simulink model "ROPOD_4Wheel_TdistZMPC_cntr_EC"  (R2017b)
settings: Solver=ode1  StartTime=0.0  StopTime=Tfinal  FixedStep=Ts  RelTol=1e-3  EnableMultiTasking=on
PreLoadFcn:
  | init_model
InitFcn:
  | init_model
values from neighbouring files (symbols this model uses):
  b_cx = 70.26    [RoPod_parameters.mat]
  b_cy = 36.5    [RoPod_parameters.mat]
  FFtheta_intia = 0    [init_model.m]
  FFxy_mass = 80    [init_model.m]
  I_fhz_dtheta_cntr = 0.5    [init_model.m]
  I_fhz_dvarphi_cntr = 0    [init_model.m]
  I_fhz_dxdy_cntr = 0.25    [init_model.m]
  k_cx = 4300    [RoPod_parameters.mat]
  k_cy = 4489    [RoPod_parameters.mat]
  K_gain_dtheta_cntr = 150    [init_model.m]
  K_gain_dvarphi_cntr = 0.05    [init_model.m]
  K_gain_dxdy_cntr = 200    [init_model.m]
  LL_wp_fhz_dtheta_cntr = 20    [init_model.m]
  LL_wp_fhz_dvarphi_cntr = 20    [init_model.m]
  LL_wp_fhz_dxdy_cntr = 20    [init_model.m]
  LL_wz_fhz_dtheta_cntr = 20    [init_model.m]
  LL_wz_fhz_dvarphi_cntr = 2    [init_model.m]
  LL_wz_fhz_dxdy_cntr = 20    [init_model.m]
  LPF_fhz_dtheta_cntr = 100    [init_model.m]
  LPF_fhz_dvarphi_cntr = 100    [init_model.m]
  LPF_fhz_dxdy_cntr = 100    [init_model.m]
  max_hw_tau = 7.0    (= 7)    [init_model.m]
  max_ropod_acc_theta = 1.6    [init_model.m]
  max_ropod_acc_xy = 1.0    (= 1)    [init_model.m]
  max_ropod_vel_theta = 1.6    [init_model.m]
  max_ropod_vel_xy = 1.0    (= 1)    [init_model.m]
  max_sw_current = 10    [init_model.m]
  Nwheels = 4    [init_model.m]
  pivot_offs_sws = [2.21 1.873 2.001 3.508]    [init_model.m]
  SW_COM1_ENABLE1 = hex2dec('0001')    [init_model.m]
  SW_COM1_ENABLE2 = hex2dec('0002')    [init_model.m]
  SW_COM1_MODE_TORQUE = bitshift(hex2dec('0000'),2)    [init_model.m]
  SW_COM1_MODE_VELOCITY = bitshift(hex2dec('0002'),2)    [init_model.m]
  SW_COM1_USE_TS = hex2dec('8000')    [init_model.m]
  sw_tau_2_curr = 1/motor_physical_parameters.torqueconstant.value    [init_model.m]
  Taucompfactor = 2.0    (= 2)    [init_model.m]
  Tinit = 1*Tslot    [init_model.m]
  Ts = 0.001    [init_model.m]
  Ts_MPC = 0.001    [init_model.m]
  xA = [1 -1 0 0 0 0 0.0206696424966 -0.0206696424966 0 0 0.0298227588181 -0.0298227588181 ... (4080 elements, 102x40)]    [ZMPCx_parameters.mat]
  xBd_dis = [1.12932348493e-06 0.000225071897401 0 0]    [ZMPCx_parameters.mat]
  xF = [0 0 0 0 0 0 0 0 0 0 0 0 ... (80 elements, 20x4)]    [ZMPCx_parameters.mat]
  xH = [20 0 0 0 0 0 0 0 0 0 0 0 ... (1600 elements, 40x40)]    [ZMPCx_parameters.mat]
  xPhi = [0.995143909015 -0.967809158823 0 0 0.980727027327 -1.91066813489 0 0 0.957042868744 -2.81984596436 0 0 ... (320 elements, 80x4)]    [ZMPCx_parameters.mat]
  xrho = 144000    [ZMPCx_parameters.mat]
  xW = [0 0 -4300 4300 0 0 -4211.12053726 4211.12053726 0 0 -4082.88267435 4082.88267435 ... (328 elements, 82x4)]    [ZMPCx_parameters.mat]
  yA = [1 -1 0 0 0 0 0.0146537039222 -0.0146537039222 0 0 0.0255124036215 -0.0255124036215 ... (4080 elements, 102x40)]    [ZMPCy_parameters.mat]
  yBd_dis = [1.24492522358e-06 0.000248362591603 0 0]    [ZMPCy_parameters.mat]
  yF = [0.00191047141222 0.00156448969707 0.00119761396088 0.000813779538874 0.00041715000072 1.20724055612e-05 -0.00039696993291 -0.000805406662726 -0.00120863105559 -0.00160205155743 -0.00198114365531 -0.00234150147928 ... (80 elements, 20x4)]    [ZMPCy_parameters.mat]
  yH = [2.00000002801 0 2.31602594113e-08 0 1.80085634996e-08 0 1.26053094289e-08 0 7.00898668547e-09 0 1.2808124932e-09 0 ... (1600 elements, 40x40)]    [ZMPCy_parameters.mat]
  yPhi = [0.994411530671 -1.11489967371 0 0 0.977778317439 -2.20691845877 0 0 0.950389393786 -3.2640842851 0 0 ... (320 elements, 80x4)]    [ZMPCy_parameters.mat]
  yrho = 10000    [ZMPCy_parameters.mat]
  yW = [0 0 -4489 4489 0 0 -4423.21952309 4423.21952309 0 0 -4308.69434324 4308.69434324 ... (328 elements, 82x4)]    [ZMPCy_parameters.mat]
undefined symbols (not defined in the file or in its folder): DiscIntNeverNeededParam, Fd_max, Fd_min, Fr_max, Fr_min, ropod_kinmodel_param
libraries: cstblocks x85, simulink x41, SOEM_EtherCAT_Lib x5
(part 5 of 5)

== stateflow chart ROPOD_4Wheel_TdistZMPC_cntr_EC/Non-ROS Ropod Controller/State machine1/Chart ==
  state Mode1_Operation_mode
    state Collision_with_object
      entry: state = 2
      state Interaction_front
        entry: ZMPC_x = 1
        entry: ZMPCx_Fd_min = 0
        entry: ZMPCx_Fd_max = Fd_max
      state Interaction_left_side
        entry: ZMPC_y = 1
        entry: ZMPCy_Fd_min = 0
        entry: ZMPCy_Fd_max = Fd_max
      state Interaction_right_side
        entry: ZMPC_y = 1
        entry: ZMPCy_Fd_min = -Fd_max
        entry: ZMPCy_Fd_max = 0
      state No_interaction
        entry: ZMPC_x = 0
        entry: ZMPC_y = 0
        entry: ZMPC_o = 0
      state Interaction_back
        entry: ZMPC_x = 1
        entry: ZMPCx_Fd_min = -Fd_max
        entry: ZMPCx_Fd_max = 0
      (default) -> Interaction_front
      Interaction_front -> Mode1_Operation_mode.Collision_with_object.No_interaction : [interaction_force_x < (Fd_min-2) ]
      Mode1_Operation_mode.Collision_with_object.No_interaction -> Interaction_front [order 3] : [interaction_force_x > (Fd_min+2)]
      Mode1_Operation_mode.Collision_with_object.No_interaction -> Mode1_Operation_mode.Collision_with_object.Interaction_left_side [order 1] : [interaction_force_y > (Fd_min+2)]
      Mode1_Operation_mode.Collision_with_object.No_interaction -> Mode1_Operation_mode.Collision_with_object.Interaction_right_side [order 2] : [interaction_force_y < -(Fd_min+2)]
      Mode1_Operation_mode.Collision_with_object.Interaction_right_side -> Mode1_Operation_mode.Collision_with_object.No_interaction : [interaction_force_y > -(Fd_min-2)]
      Mode1_Operation_mode.Collision_with_object.Interaction_left_side -> Mode1_Operation_mode.Collision_with_object.No_interaction : [interaction_force_y < (Fd_min-2) ]
      Mode1_Operation_mode.Collision_with_object.No_interaction -> Interaction_back [order 4] : [interaction_force_x < -(Fd_min+2)]
      Interaction_back -> Mode1_Operation_mode.Collision_with_object.No_interaction : [interaction_force_x > -(Fd_min-2)]
    state Interaction_left_side
      entry: state = 3
      entry: ZMPC_y = 1
      entry: ZMPCy_Fd_min = 0
      entry: ZMPCy_Fd_max = Fd_max
    state Interaction_right_side
      entry: state = 3
      entry: ZMPC_y = 1
      entry: ZMPCy_Fd_min = -Fd_max
      entry: ZMPCy_Fd_max = 0
    state No_interaction
      entry: state = 1
      entry: ZMPC_x = 0
      entry: ZMPC_y = 0
      entry: ZMPC_o = 0
    Mode1_Operation_mode.Interaction_left_side -> Collision_with_object [order 2] : [interaction_force_x > Fd_min]
    Mode1_Operation_mode.No_interaction -> Collision_with_object [order 1] : [interaction_force_x > Fd_min]
    Mode1_Operation_mode.Interaction_right_side -> Collision_with_object [order 2] : [interaction_force_x > Fd_min]
    Mode1_Operation_mode.No_interaction -> Mode1_Operation_mode.Interaction_left_side [order 2] : [interaction_force_y > (Fd_min+2)]
    Mode1_Operation_mode.No_interaction -> Mode1_Operation_mode.Interaction_right_side [order 3] : [interaction_force_y < -(Fd_min+2)]
    Mode1_Operation_mode.Interaction_right_side -> Mode1_Operation_mode.No_interaction [order 1] : [interaction_force_y > -(Fd_min-2)]
    Mode1_Operation_mode.Interaction_left_side -> Mode1_Operation_mode.No_interaction [order 1] : [interaction_force_y < (Fd_min-2) ]
    (default) -> Mode1_Operation_mode.No_interaction
  state Mode4_Connect_to_cart
    state Connect_to_cart
      entry: ZMPC_x = 0
      entry: ZMPC_y = 0
      entry: ZMPC_o = 0
    state Hold_contact_with_cart
      entry: state = 4
      entry: ZMPC_x = 1
      entry: ZMPC_o = 1
      entry: ZMPCx_Fd_min = -Fd_max
      entry: ZMPCx_Fd_max = -Fd_min
    (default) -> Connect_to_cart
    Hold_contact_with_cart -> Connect_to_cart : [interaction_force_x > -(Fd_min-7)]
    Connect_to_cart -> Hold_contact_with_cart : [interaction_force_x < -(Fd_min+2)]
  state Velocity_control
    entry: state = 0
    entry: ZMPC_x = 0
    entry: ZMPC_y = 0
    entry: ZMPC_o = 0
    entry: ZMPCx_Fd_min = 0
    entry: ZMPCx_Fd_max = Fd_max
    entry: ZMPCy_Fd_min = 0
    entry: ZMPCy_Fd_max = Fd_max
  (default) -> Velocity_control
  Velocity_control -> Mode1_Operation_mode : [mode == 1]
  Mode1_Operation_mode -> Mode4_Connect_to_cart : [mode == 4]
  Collision_with_object -> Velocity_control : [mode == 0]
  Mode4_Connect_to_cart -> Mode1_Operation_mode : [mode == 1]
  data: interaction_force_x input; ZMPC_x output; ZMPC_y output; ZMPC_o output; interaction_force_y input; Fd_min input; ZMPCx_Fd_min output; ZMPCy_Fd_min output; Fd_max input; ZMPCx_Fd_max output; ZMPCy_Fd_max output; state output; mode input

== matlab function ROPOD_4Wheel_TdistZMPC_cntr_EC/Non-ROS Ropod Controller/platform vel cntr/Bumper Interaction Controller/Bumper_system/cal1/Calibration1 ==
  data: angle input; cal_angle output; sample input; i output; data input; data_out output
function [cal_angle, i, data_out]= fcn(angle,sample,data)
cal_start_sample = 1000;
cal_end_sample = 2000;

if sample > cal_start_sample && sample <= cal_end_sample
    data_out = data+angle; 
    cal_angle = angle;
else
    correction = data/(cal_end_sample - cal_start_sample);
    cal_angle = angle-correction;
    data_out = data;
end

i = sample+1;

== matlab function ROPOD_4Wheel_TdistZMPC_cntr_EC/Non-ROS Ropod Controller/platform vel cntr/Bumper Interaction Controller/Bumper_system/cal2/Calibration1 ==
  data: angle input; cal_angle output; sample input; i output; data input; data_out output
function [cal_angle, i, data_out]= fcn(angle,sample,data)
cal_start_sample = 1000;
cal_end_sample = 2000;

if sample > cal_start_sample && sample <= cal_end_sample
    data_out = data+angle; 
    cal_angle = angle;
else
    correction = data/(cal_end_sample - cal_start_sample);
    cal_angle = angle-correction;
    data_out = data;
end

i = sample+1;

== matlab function ROPOD_4Wheel_TdistZMPC_cntr_EC/Non-ROS Ropod Controller/platform vel cntr/Bumper Interaction Controller/Bumper_system/cal3/Calibration1 ==
  data: angle input; cal_angle output; sample input; i output; data input; data_out output
function [cal_angle, i, data_out]= fcn(angle,sample,data)
cal_start_sample = 1000;
cal_end_sample = 2000;

if sample > cal_start_sample && sample <= cal_end_sample
    data_out = data+angle; 
    cal_angle = angle;
else
    correction = data/(cal_end_sample - cal_start_sample);
    cal_angle = angle-correction;
    data_out = data;
end

i = sample+1;

== matlab function ROPOD_4Wheel_TdistZMPC_cntr_EC/Non-ROS Ropod Controller/platform vel cntr/Bumper Interaction Controller/Bumper_system/cal4/Calibration1 ==
  data: angle input; cal_angle output; sample input; i output; data input; data_out output
function [cal_angle, i, data_out]= fcn(angle,sample,data)
cal_start_sample = 1000;
cal_end_sample = 2000;

if sample > cal_start_sample && sample <= cal_end_sample
    data_out = data+angle; 
    cal_angle = angle;
else
    correction = data/(cal_end_sample - cal_start_sample);
    cal_angle = angle-correction;
    data_out = data;
end

i = sample+1;

== matlab function ROPOD_4Wheel_TdistZMPC_cntr_EC/Non-ROS Ropod Controller/platform vel cntr/Bumper Interaction Controller/Bumper_system/cal5/Calibration1 ==
  data: angle input; cal_angle output; sample input; i output; data input; data_out output
function [cal_angle, i, data_out]= fcn(angle,sample,data)
cal_start_sample = 1000;
cal_end_sample = 2000;

if sample > cal_start_sample && sample <= cal_end_sample
    data_out = data+angle; 
    cal_angle = angle;
else
    correction = data/(cal_end_sample - cal_start_sample);
    cal_angle = angle-correction;
    data_out = data;
end

i = sample+1;

== matlab function ROPOD_4Wheel_TdistZMPC_cntr_EC/Non-ROS Ropod Controller/platform vel cntr/Bumper Interaction Controller/Bumper_system/cal6/Calibration1 ==
  data: angle input; cal_angle output; sample input; i output; data input; data_out output
function [cal_angle, i, data_out]= fcn(angle,sample,data)
cal_start_sample = 1000;
cal_end_sample = 2000;

if sample > cal_start_sample && sample <= cal_end_sample
    data_out = data+angle; 
    cal_angle = angle;
else
    correction = data/(cal_end_sample - cal_start_sample);
    cal_angle = angle-correction;
    data_out = data;
end

i = sample+1;

== matlab function ROPOD_4Wheel_TdistZMPC_cntr_EC/Non-ROS Ropod Controller/platform vel cntr/Bumper Interaction Controller/Bumper_system/cal7/Calibration1 ==
  data: angle input; cal_angle output; sample input; i output; data input; data_out output
function [cal_angle, i, data_out]= fcn(angle,sample,data)
cal_start_sample = 1000;
cal_end_sample = 2000;

if sample > cal_start_sample && sample <= cal_end_sample
    data_out = data+angle; 
    cal_angle = angle;
else
    correction = data/(cal_end_sample - cal_start_sample);
    cal_angle = angle-correction;
    data_out = data;
end

i = sample+1;

== stateflow chart ROPOD_4Wheel_TdistZMPC_cntr_EC/joystick_velocitie_sp/Chart ==
  state init
    entry: velocity_sp = [0; 0; 0]
  state Wait_for_joystick_command
    entry: mode = 0
    entry: velocity_sp = [0; 0; 0]
  state idle [commented out]
    entry: mode = 0
  state Move_right
    entry: velocity_sp = [0; -0.4; 0]
  state Rotate_left
    entry: velocity_sp = [0; 0; 0.4]
  state Rotate_right
    entry: velocity_sp = [0; 0; -0.4]
  state Move_back
    entry: mode = 1
  state Move_backward
    entry: velocity_sp = [-0.4; 0; 0]
  state Move_left
    entry: velocity_sp = [0; 0.4; 0]
  state Move_forward
    entry: mode = 1
    entry: velocity_sp = [0.4; 0; 0]
  state Connect_to_cart
    entry: connected_to_cart = 0
    entry: mode = 4
    entry: velocity_sp = [-0.3; 0; 0]
  state Connected_to_cart
    entry: velocity_sp = [0; 0; 0]
    entry: connected_to_cart = 1
  (default) -> init
  init -> Wait_for_joystick_command : after(3,sec)
  Wait_for_joystick_command -> idle [commented out] : [robot_speed(1) < 0.02 && robot_speed(1) > -0.02 && robot_speed(2) < 0.02 && robot_speed(2) > -0.02 && robot_speed(3) < 0.02 && robot_speed(3) > -0.02]
  idle -> Wait_for_joystick_command [commented out] : [joystick ~= 0]
  Wait_for_joystick_command -> Move_forward [order 3] : [joystick == 1]
  Move_forward -> Wait_for_joystick_command : [joystick ~= 1]
  Wait_for_joystick_command -> Move_backward [order 2] : [joystick == 2]
  Move_backward -> Wait_for_joystick_command : [joystick ~= 2]
  Wait_for_joystick_command -> Move_left [order 6] : [joystick == 3]
  Move_left -> Wait_for_joystick_command : [joystick ~= 3]
  Wait_for_joystick_command -> Move_right [order 5] : [joystick == 4]
  Move_right -> Wait_for_joystick_command : [joystick ~= 4]
  Rotate_left -> Wait_for_joystick_command : [joystick ~= 8]
  Wait_for_joystick_command -> Rotate_left [order 7] : [joystick == 8]
  Rotate_right -> Wait_for_joystick_command : [joystick ~= 9]
  Wait_for_joystick_command -> Rotate_right [order 4] : [joystick == 9]
  Connected_to_cart -> Wait_for_joystick_command
  Move_back -> Wait_for_joystick_command [order 1] : [joystick ~= 12]
  Wait_for_joystick_command -> Move_back [order 1] : [joystick == 12]
  Move_back -> Connect_to_cart [order 2] : [after(0.1,sec)]
  Connect_to_cart -> Connected_to_cart : [Fx_Fy_Tx_Ty(1) > 30 && joystick ~= 12]
  data: joystick input; velocity_sp output; robot_speed input; mode output; Fx_Fy_Tx_Ty input; connected_to_cart output

== matlab function ROPOD_4Wheel_TdistZMPC_cntr_EC/Non-ROS Ropod Controller/platform vel cntr/Bumper Interaction Controller/Bumper_system/cal8/Calibration1 ==
  data: angle input; cal_angle output; sample input; i output; data input; data_out output
function [cal_angle, i, data_out]= fcn(angle,sample,data)
cal_start_sample = 1000;
cal_end_sample = 2000;

if sample > cal_start_sample && sample <= cal_end_sample
    data_out = data+angle; 
    cal_angle = angle;
else
    correction = data/(cal_end_sample - cal_start_sample);
    cal_angle = angle-correction;
    data_out = data;
end

i = sample+1;

== matlab function ROPOD_4Wheel_TdistZMPC_cntr_EC/Non-ROS Ropod Controller/platform vel cntr/Bumper Interaction Controller/Bumper_system/speed deflection angle calculation X+ ==
  data: s_data input; Total_deflection output; Total_speed output; max_angle output
function [Total_deflection, Total_speed, max_angle] = Sensor_data(s_data)
% s_data is the sensor data
% s_data(1:4) = deflection in m
% s_data(5:8) = speed in m/s

% Parameters

%               V end-effector V            %
%-------------------------------------------%
% .            .             .            . %
% .            .             .            . %
%_I_          _I_           _I_          _I_%
% <     d1    ><     d2     ><      d3    > %
% x1          x2            x3           x4 %

d1 = 164; %mm
d2 = 164; %mm 
d3 = 164; %mm
dx = s_data(1:4); %deflection in m
dx_dot = s_data(5:8); %speed in m/s


% Deflection and speed in x direction
Total_deflection = sum(dx);
Total_speed = sum(dx_dot);


% Angle of the end-effector
angle_12 = atan((dx(1)-dx(2))/(d1));
angle_23 = atan((dx(2)-dx(3))/(d2));
angle_34 = atan((dx(3)-dx(4))/(d3));
angle_14 = atan((dx(1)-dx(4))/(d1+d2+d3));
angle = max([angle_12, angle_23, angle_34, angle_14]);
max_angle = rad2deg(angle);

end

== matlab function ROPOD_4Wheel_TdistZMPC_cntr_EC/Non-ROS Ropod Controller/platform vel cntr/Bumper Interaction Controller/Bumper_system/speed deflection angle calculation X- ==
  data: s_data input; Total_deflection output; Total_speed output; max_angle output
function [Total_deflection, Total_speed, max_angle] = Sensor_data(s_data)
% s_data is the sensor data
% s_data(1:4) = deflection in m
% s_data(5:8) = speed in m/s

% Parameters

%               V end-effector V            %
%-------------------------------------------%
% .            .             .            . %
% .            .             .            . %
%_I_          _I_           _I_          _I_%
% <     d1    ><     d2     ><      d3    > %
% x1          x2            x3           x4 %

d1 = 164; %mm
d2 = 164; %mm 
d3 = 164; %mm
dx = s_data(1:4); %deflection in m
dx_dot = s_data(5:8); %speed in m/s


% Deflection and speed in x direction
Total_deflection = sum(dx);
Total_speed = sum(dx_dot);


% Angle of the end-effector
angle_12 = atan((dx(1)-dx(2))/(d1));
angle_23 = atan((dx(2)-dx(3))/(d2));
angle_34 = atan((dx(3)-dx(4))/(d3));
angle_14 = atan((dx(1)-dx(4))/(d1+d2+d3));
angle = max([angle_12, angle_23, angle_34, angle_14]);
max_angle = rad2deg(angle);

end

== matlab function ROPOD_4Wheel_TdistZMPC_cntr_EC/Non-ROS Ropod Controller/platform vel cntr/Bumper Interaction Controller/Bumper_system/speed deflection angle calculation Y+ ==
  data: s_data input; Total_deflection output; Total_speed output; max_angle output
function [Total_deflection, Total_speed, max_angle] = Sensor_data(s_data)
% s_data is the sensor data
% s_data(1:4) = deflection in m
% s_data(5:8) = speed in m/s

% Parameters

%               V end-effector V            %
%-------------------------------------------%
% .            .             .            . %
% .            .             .            . %
%_I_          _I_           _I_          _I_%
% <     d1    ><     d2     ><      d3    > %
% x1          x2            x3           x4 %

d1 = 164; %mm
d2 = 164; %mm 
d3 = 164; %mm
dx = s_data(1:4); %deflection in m
dx_dot = s_data(5:8); %speed in m/s


% Deflection and speed in x direction
Total_deflection = sum(dx);
Total_speed = sum(dx_dot);


% Angle of the end-effector
angle_12 = atan((dx(1)-dx(2))/(d1));
angle_23 = atan((dx(2)-dx(3))/(d2));
angle_34 = atan((dx(3)-dx(4))/(d3));
angle_14 = atan((dx(1)-dx(4))/(d1+d2+d3));
angle = max([angle_12, angle_23, angle_34, angle_14]);
max_angle = rad2deg(angle);

end

== matlab function ROPOD_4Wheel_TdistZMPC_cntr_EC/Non-ROS Ropod Controller/platform vel cntr/Bumper Interaction Controller/Bumper_system/speed deflection angle calculation Y- ==
  data: s_data input; Total_deflection output; Total_speed output; max_angle output
function [Total_deflection, Total_speed, max_angle] = Sensor_data(s_data)
% s_data is the sensor data
% s_data(1:4) = deflection in m
% s_data(5:8) = speed in m/s

% Parameters

%               V end-effector V            %
%-------------------------------------------%
% .            .             .            . %
% .            .             .            . %
%_I_          _I_           _I_          _I_%
% <     d1    ><     d2     ><      d3    > %
% x1          x2            x3           x4 %

d1 = 164; %mm
d2 = 164; %mm 
d3 = 164; %mm
dx = s_data(1:4); %deflection in m
dx_dot = s_data(5:8); %speed in m/s


% Deflection and speed in x direction
Total_deflection = sum(dx);
Total_speed = sum(dx_dot);


% Angle of the end-effector
angle_12 = atan((dx(1)-dx(2))/(d1));
angle_23 = atan((dx(2)-dx(3))/(d2));
angle_34 = atan((dx(3)-dx(4))/(d3));
angle_14 = atan((dx(1)-dx(4))/(d1+d2+d3));
angle = max([angle_12, angle_23, angle_34, angle_14]);
max_angle = rad2deg(angle);

end

== matlab function ROPOD_4Wheel_TdistZMPC_cntr_EC/Non-ROS Ropod Controller/platform vel cntr/Bumper Interaction Controller/ZMPC_x/Zone MPC ==
  data: epsilon output; u_f output size=1; mo input size=4; Fd_max input; Fd_min input; Fr_max input; Fr_min input; Bd_dis input; H input; F input; A input; W input; Phi input; rho input; epsilon_old input; uf_old input; mv_old input; exitflag_old input; mv output; exitflag output; iA0 input; iA output; s_old input; s output size=1
function [epsilon, u_f, mv, exitflag, iA, s] = Zone_MPC(mo, Fd_max, Fd_min, Fr_max, Fr_min, Bd_dis, H, F, A, W, Phi, rho, epsilon_old, uf_old, mv_old, exitflag_old, iA0, s_old)
% mv is controller output
% mo is the feedback of the states
% ref is not used
% md is measured disturbance

%% Sample time of 0.01 (10 times slower)
s = s_old;
if s == 10

%% Precalculated matrices 
N = 20;

%% getWLc
Xmax = Fd_max;
Xmin = Fd_min;
umax = Fr_max;
umin = Fr_min;

n = size(Phi,1)/size(Bd_dis,1);
bi = [umax;
      -umin; 
      Xmax;
      -Xmin];

bN = [Xmax;
     -Xmin];

c = zeros(length(bi)*n+length(bN),1);
r_size = size(bi,1);
for i = 1:n 
    c((i-1)*r_size+1:i*r_size,1) = bi;
end
c(size(c,1)+1-size(bN,1):size(c,1),1) = bN;

%%
if iA0 == 0.0
    iA0 = false(size([W*[0; 0; 0; 0]+c;zeros(N,1)]));
else
    iA0 = logical(iA0);
end
LL = chol(H, 'lower');
Linv = LL\eye(size(H,1));
opt = mpcqpsolverOptions;
opt.IntegrityChecks = false;

%% f matrix
xk = mo;
Fxk = F*xk;
f = zeros(N*2,1);
i = 1;
j = 1;
k = 2;
while i <= N
    f(j,1) = Fxk(i,1);
    f(k,1) = rho;
    i = i+1;
    j = j+2;
    k = k+2;
end

%% solve qp problem
[u_qp, exitflag, iAi] = mpcqpsolver(Linv, f, -A, -([W*xk+c;zeros(N,1)]), [], zeros(0,1), iA0, opt);
mv = 0.0;
u_mpc = u_qp(1);
epsilon = u_qp(2);

%% Friction compensation
% xkp1 = Ad_dis*xk+Bd_dis*u_qp(1);
% v = xkp1(2);
% 
% F_brk = 43.6;
% F_c = 26.16;
% f = 1.12;
% v_brk = 0.05;
% 
% v_st = v_brk*sqrt(2);
% v_coul = v_brk/10;
% u_f = sqrt(2*exp(1))*(F_brk-F_c)*exp(-(v/v_st)^2)*v/v_st+F_c*tanh(v/v_coul)+v*f;
u_f = 0;%%%%%%!!!!!!!!!!!!!!!


%% Output
mv = u_mpc + u_f;
iA = double(iAi);
s = 1;

else 
    %Neuspeuteren
    epsilon = epsilon_old;
    u_f = uf_old;
    mv = mv_old;
    exitflag = exitflag_old;
    iA = iA0; %!!!!!!!!!!!
    s = s+1;    
end

end

== matlab function ROPOD_4Wheel_TdistZMPC_cntr_EC/Non-ROS Ropod Controller/platform vel cntr/Bumper Interaction Controller/ZMPC_y/Zone MPC ==
  data: epsilon output; u_f output size=1; mo input size=4; Fd_max input; Fd_min input; Fr_max input; Fr_min input; Bd_dis input; H input; F input; A input; W input; Phi input; rho input; epsilon_old input; uf_old input; mv_old input; exitflag_old input; mv output; exitflag output; iA0 input; iA output; s_old input; s output size=1
function [epsilon, u_f, mv, exitflag, iA, s] = Zone_MPC(mo, Fd_max, Fd_min, Fr_max, Fr_min, Bd_dis, H, F, A, W, Phi, rho, epsilon_old, uf_old, mv_old, exitflag_old, iA0, s_old)
% mv is controller output
% mo is the feedback of the states
% ref is not used
% md is measured disturbance

%% Sample time of 0.01 (10 times slower)
s = s_old;
if s == 10

%% Precalculated matrices 
N = 20;

%% getWLc
Xmax = Fd_max;
Xmin = Fd_min;
umax = Fr_max;
umin = Fr_min;

n = size(Phi,1)/size(Bd_dis,1);
bi = [umax;
      -umin; 
      Xmax;
      -Xmin];

bN = [Xmax;
     -Xmin];

c = zeros(length(bi)*n+length(bN),1);
r_size = size(bi,1);
for i = 1:n 
    c((i-1)*r_size+1:i*r_size,1) = bi;
end
c(size(c,1)+1-size(bN,1):size(c,1),1) = bN;

%%
if iA0 == 0.0
    iA0 = false(size([W*[0; 0; 0; 0]+c;zeros(N,1)]));
else
    iA0 = logical(iA0);
end
LL = chol(H, 'lower');
Linv = LL\eye(size(H,1));
opt = mpcqpsolverOptions;
opt.IntegrityChecks = false;

%% f matrix
xk = mo;
Fxk = F*xk;
f = zeros(N*2,1);
i = 1;
j = 1;
k = 2;
while i <= N
    f(j,1) = Fxk(i,1);
    f(k,1) = rho;
    i = i+1;
    j = j+2;
    k = k+2;
end

%% solve qp problem
[u_qp, exitflag, iAi] = mpcqpsolver(Linv, f, -A, -([W*xk+c;zeros(N,1)]), [], zeros(0,1), iA0, opt);
mv = 0.0;
u_mpc = u_qp(1);
epsilon = u_qp(2);

%% Friction compensation
% xkp1 = Ad_dis*xk+Bd_dis*u_qp(1);
% v = xkp1(2);
% 
% F_brk = 43.6;
% F_c = 26.16;
% f = 1.12;
% v_brk = 0.05;
% 
% v_st = v_brk*sqrt(2);
% v_coul = v_brk/10;
% u_f = sqrt(2*exp(1))*(F_brk-F_c)*exp(-(v/v_st)^2)*v/v_st+F_c*tanh(v/v_coul)+v*f;
u_f = 0;%%%%%%!!!!!!!!!!!!!!!


%% Output
mv = u_mpc + u_f;
iA = double(iAi);
s = 1;

else 
    %Neuspeuteren
    epsilon = epsilon_old;
    u_f = uf_old;
    mv = mv_old;
    exitflag = exitflag_old;
    iA = iA0; %!!!!!!!!!!!
    s = s+1;    
end

end

== matlab function ROPOD_4Wheel_TdistZMPC_cntr_EC/Non-ROS Ropod Controller/platform vel cntr/Inverse Kinematics 4SW/Gl_matrix ==
  data: ropod_kinmodel_param_vec input; Gl output; delta input
function Gl = Gl_matrix_wrapper(ropod_kinmodel_param_vec, delta)

Gl = Gl_matrix_wrapper(ropod_kinmodel_param_vec, delta);

end

== matlab function ROPOD_4Wheel_TdistZMPC_cntr_EC/Non-ROS Ropod Controller/platform vel cntr/Torque distribution/Gl_matrices ==
  data: ropod_kinmodel_param_vec input; Gl output; delta input; Gtl output; GtSl output
function [Gl, Gtl, GtSl]   = G_matrices( ropod_kinmodel_param_vec, delta)
%ROPOD_JACOBIAN Summary of this function goes here
%   Detailed explanation goes here


Gl    = Gl_matrix_wrapper(ropod_kinmodel_param_vec, delta);
Gtl   = Gl.';
GtSl  = Gtl*S_matrix();
end

== matlab function ROPOD_4Wheel_TdistZMPC_cntr_EC/Non-ROS Ropod Controller/platform vel cntr/Torque distribution/platform_forces_2_tau_dist_optimal ==
  data: GtSl input; taubody input; ena_w input; Ttaud output; tau_max input; taubody_sc output
function [Ttaud, taubody_sc]   = Ttaud_optimal_vec( GtSl, taubody, ena_w , tau_max)
%#codegen

[Ttaud, taubody_sc]   = tau_optimal_dist_vec_fun( GtSl, taubody, ena_w, tau_max);

end

== matlab function ROPOD_4Wheel_TdistZMPC_cntr_EC/Non-ROS Ropod Controller/wheel flip compensation/MATLAB Function ==
  data: tl input; tl_out output; tr input; ropod_kinmodel_param_vec input size=18; tr_out output; kmax input; sc output
function [tl_out,tr_out, sc] = fcn(tl, tr, ropod_kinmodel_param_vec, kmax)

[  rW1_1,rW1_2,rW1_3,rW1_4,rW2_1,rW2_2,rW2_3,rW2_4,...
    s_w,...
    d_w, ...
    CW1_1,CW1_2,CW1_3,CW1_4,CW2_1,CW2_2,CW2_3,CW2_4 ...
    ]= extract_kinmodel_parameters(ropod_kinmodel_param_vec);

Fxi = (tl/rW1_1+tr/rW1_2);
Fyi = (tr/rW1_2-tl/rW1_1)*(d_w/(2*s_w));
theta = atan2(Fyi,Fxi);

Fsize = sqrt(Fxi*Fxi+Fyi*Fyi);
if Fsize> 30
   sc = (1+(kmax-1)*abs(sin(theta)));
else
    sc = 1;
end

tl_out = tl*sc;
tr_out = tr*sc;

== matlab function ROPOD_4Wheel_TdistZMPC_cntr_EC/Non-ROS Ropod Controller/wheel flip compensation/MATLAB Function1 ==
  data: tl input; tl_out output; tr input; ropod_kinmodel_param_vec input size=18; tr_out output; kmax input
function [tl_out,tr_out] = fcn(tl, tr, ropod_kinmodel_param_vec, kmax)

[  rW1_1,rW1_2,rW1_3,rW1_4,rW2_1,rW2_2,rW2_3,rW2_4,...
    s_w,...
    d_w, ...
    CW1_1,CW1_2,CW1_3,CW1_4,CW2_1,CW2_2,CW2_3,CW2_4 ...
    ]= extract_kinmodel_parameters(ropod_kinmodel_param_vec);

Fxi = (tl/rW1_1+tr/rW1_2);
Fyi = (tr/rW1_2-tl/rW1_1)*(d_w/(2*s_w));
theta = atan2(Fyi,Fxi);

Fsize = sqrt(Fxi*Fxi+Fyi*Fyi);
if Fsize> 30
   sc = (1+(kmax-1)*abs(sin(theta)));
else
    sc = 1;
end

tl_out = tl*sc;
tr_out = tr*sc;

== matlab function ROPOD_4Wheel_TdistZMPC_cntr_EC/Non-ROS Ropod Controller/wheel flip compensation/MATLAB Function2 ==
  data: tl input; tl_out output; tr input; ropod_kinmodel_param_vec input size=18; tr_out output; kmax input
function [tl_out,tr_out] = fcn(tl, tr, ropod_kinmodel_param_vec, kmax)

[  rW1_1,rW1_2,rW1_3,rW1_4,rW2_1,rW2_2,rW2_3,rW2_4,...
    s_w,...
    d_w, ...
    CW1_1,CW1_2,CW1_3,CW1_4,CW2_1,CW2_2,CW2_3,CW2_4 ...
    ]= extract_kinmodel_parameters(ropod_kinmodel_param_vec);

Fxi = (tl/rW1_1+tr/rW1_2);
Fyi = (tr/rW1_2-tl/rW1_1)*(d_w/(2*s_w));
theta = atan2(Fyi,Fxi);

Fsize = sqrt(Fxi*Fxi+Fyi*Fyi);
if Fsize> 30
   sc = (1+(kmax-1)*abs(sin(theta)));
else
    sc = 1;
end

tl_out = tl*sc;
tr_out = tr*sc;

== matlab function ROPOD_4Wheel_TdistZMPC_cntr_EC/Non-ROS Ropod Controller/wheel flip compensation/MATLAB Function3 ==
  data: tl input; tl_out output; tr input; ropod_kinmodel_param_vec input size=18; tr_out output; kmax input
function [tl_out,tr_out] = fcn(tl, tr, ropod_kinmodel_param_vec, kmax)

[  rW1_1,rW1_2,rW1_3,rW1_4,rW2_1,rW2_2,rW2_3,rW2_4,...
    s_w,...
    d_w, ...
    CW1_1,CW1_2,CW1_3,CW1_4,CW2_1,CW2_2,CW2_3,CW2_4 ...
    ]= extract_kinmodel_parameters(ropod_kinmodel_param_vec);

Fxi = (tl/rW1_1+tr/rW1_2);
Fyi = (tr/rW1_2-tl/rW1_1)*(d_w/(2*s_w));
theta = atan2(Fyi,Fxi);

Fsize = sqrt(Fxi*Fxi+Fyi*Fyi);
if Fsize> 30
   sc = (1+(kmax-1)*abs(sin(theta)));
else
    sc = 1;
end

tl_out = tl*sc;
tr_out = tr*sc;
